simulink model "Modelo_benchmark"  (R2023a)
settings: Solver=VariableStepAuto  StartTime=0.0  StopTime=6250  RelTol=1e-3
values from neighbouring files (symbols this model uses):
  A = 0.0012    [control_temperatura.mat]    (also in var.m)
  C1_Q1 = 64.8931891795    [control_temperatura.mat]    (also in var.m = k3*Tau2)
  C1_Q2 = 0.0892445260493    [control_temperatura.mat]    (also in var.m = k1*k6)
  C2_Q1 = 0.558623321055    [control_temperatura.mat]    (also in var.m = k3)
  C_ff = GQ2T1cr/GQ1T1cr    [var.m]
  cp = 500    [control_temperatura.mat]    (also in var.m)
  e = zeros(1,iteraciones+ini)    [Codigo_discreto_ap.m]    (also in control_temperatura.mat = 0.9; var.m = 0.9)
  GQ1T1cr = tf(kcr1, [Taucr1 1])    [var.m]
  Hf1 = 0.01    [control_temperatura.mat]    (also in var.m)
  Hf2 = 0.004    [control_temperatura.mat]    (also in var.m)
  K_ap = 7.31538861094    [control_temperatura.mat]    (also in var.m = (2*delta*Taucr1*wn-1)/kcr1)
  K_cp = 1.15885597738    [control_temperatura.mat]    (also in var.m)
  m = 0.004    [control_temperatura.mat]    (also in var.m)
  P1_Q1 = 12978.6378359    [control_temperatura.mat]    (also in var.m = Tau1*Tau2)
  P1_Q2 = 12978.6378359    [control_temperatura.mat]    (also in var.m = Tau1*Tau2)
  P2_Q1 = 227.890937142    [control_temperatura.mat]    (also in var.m = Tau2+Tau1)
  P2_Q2 = 227.890937142    [control_temperatura.mat]    (also in var.m = Tau2+Tau1)
  P3_Q1 = 0.840856230771    [control_temperatura.mat]    (also in var.m = 1- k1*k4)
  P3_Q2 = 0.840856230771    [control_temperatura.mat]    (also in var.m = 1- k1*k4)
  T1i = 299.55    [control_temperatura.mat]    (also in var.m)
  T1o = 309.62355074    [control_temperatura.mat]    (also in var.m = x(1))
  T2i = 299.55    [control_temperatura.mat]    (also in var.m)
  TA = 299.55    [control_temperatura.mat]    (also in var.m)
  th = 5.67e-08    [control_temperatura.mat]    (also in var.m)
  Ti_ap = 23.6710802631    [control_temperatura.mat]    (also in var.m = (K_ap*kcr1)/(Taucr1*wn^2))
  Ti_cp = 165    [control_temperatura.mat]    (also in var.m)
  Tk = 273.15    [control_temperatura.mat]    (also in var.m)
  Tt_ap = 4.8652934406    [control_temperatura.mat]    (also in var.m = sqrt(Ti_ap))
  Tt_cp = 12.8452325787    [control_temperatura.mat]    (also in var.m = sqrt(Ti_cp))
  U = 1.4    [control_temperatura.mat]    (also in var.m)
undefined symbols (not defined in the file or in its folder): PID_Matlab
libraries: slpidlib x8, simulink_extras x6, simulink x4
(part 2 of 2)

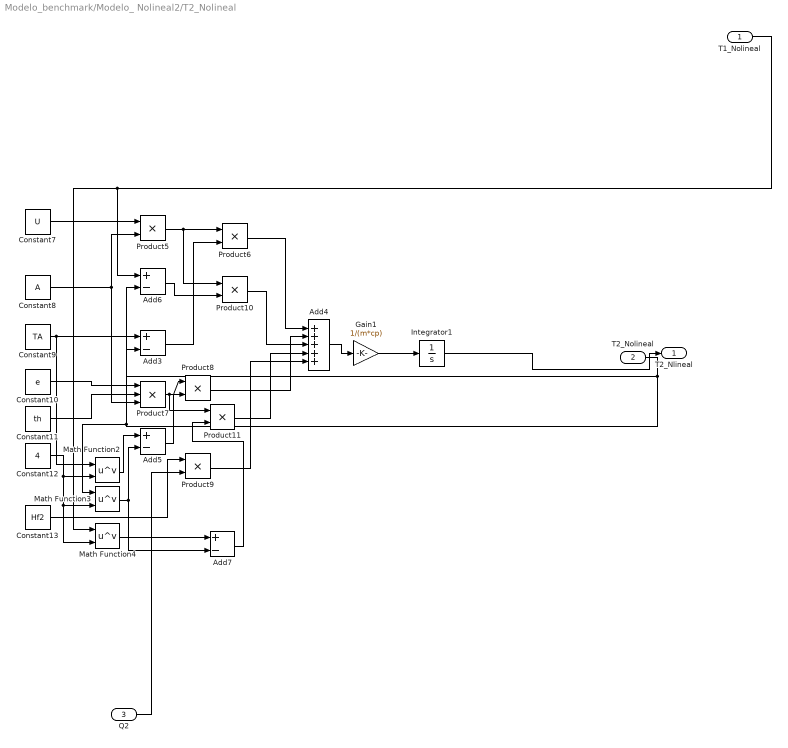
== system Modelo_benchmark/Modelo_ Nolineal2/T2_Nolineal ==
  T1_Nolineal : Inport
  T2_Nolineal : Inport  Port=2
  Q2 : Inport  Port=3
  Add{3,5..7} (4 alike) : Sum  Inputs=+-
  Add4 : Sum  Inputs=+++++
  Constant10 : Constant  Value=e
  Constant11 : Constant  Value=th
  Constant12 : Constant  Value=4
  Constant13 : Constant  Value=Hf2
  Constant7 : Constant  Value=U
  Constant8 : Constant  Value=A
  Constant9 : Constant  Value=TA
  Gain1 : Gain  Gain=1/(m*cp)
  Integrator1 : Integrator  InitialCondition=T2i
  Math Function2 : Math  Operator=pow
  Math Function3 : Math  Operator=pow
  Math Function4 : Math  Operator=pow
  Product{5..6,8..11} (6 alike) : Product
  Product7 : Product  Inputs=3
  T2_Nlineal : Outport
  wires:
  Integrator1/1 -> T2_Nlineal/1
  Product11/1 -> Add4/4
  T2_Nolineal/1 -> Add3/2, Math Function3/1, Add6/2
  Product7/1 -> Product11/1, Product8/1
  Constant7/1 -> Product5/1
  Product8/1 -> Add4/2
  T1_Nolineal/1 -> Math Function4/1, Add6/1
  Product9/1 -> Add4/5
  Math Function3/1 -> Add7/2, Add5/2
  Add6/1 -> Product10/2
  Add3/1 -> Product6/2
  Constant9/1 -> Math Function2/1, Add3/1
  Constant12/1 -> Math Function4/2, Math Function3/2, Math Function2/2
  Add4/1 -> Gain1/1
  Add5/1 -> Product8/2
  Constant11/1 -> Product7/2
  Constant13/1 -> Product9/1
  Gain1/1 -> Integrator1/1
  Constant8/1 -> Product5/2, Product7/3
  Product10/1 -> Add4/3
  Math Function4/1 -> Add7/1
  Math Function2/1 -> Add5/1
  Product6/1 -> Add4/1
  Q2/1 -> Product9/2
  Constant10/1 -> Product7/1
  Product5/1 -> Product10/1, Product6/1
  Add7/1 -> Product11/2

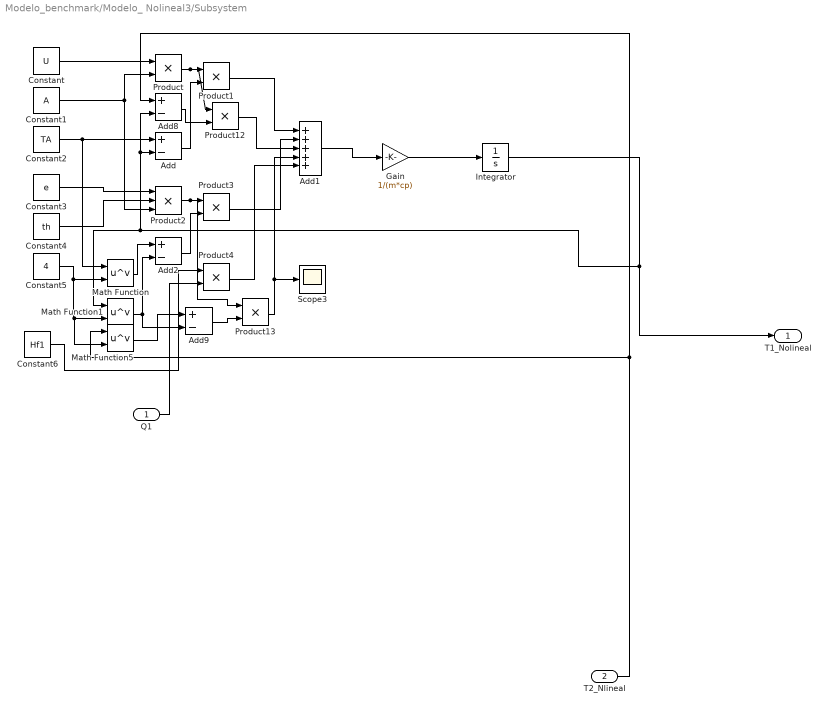
== system Modelo_benchmark/Modelo_ Nolineal3/Subsystem ==
  Q1 : Inport
  T2_Nlineal : Inport  Port=2
  Add{,2,8..9} (4 alike) : Sum  Inputs=+-
  Add1 : Sum  Inputs=+++++
  Constant : Constant  Value=U
  Constant1 : Constant  Value=A
  Constant2 : Constant  Value=TA
  Constant3 : Constant  Value=e
  Constant4 : Constant  Value=th
  Constant5 : Constant  Value=4
  Constant6 : Constant  Value=Hf1
  Gain : Gain  Gain=1/(m*cp)
  Integrator : Integrator  InitialCondition=T1i
  Math Function : Math  Operator=pow
  Math Function1 : Math  Operator=pow
  Math Function5 : Math  Operator=pow
  Product{,1,3..4,12..13} (6 alike) : Product
  Product2 : Product  Inputs=3
  Scope3 : Scope
  T1_Nolineal : Outport
  wires:
  Add/1 -> Product1/2
  Constant4/1 -> Product2/2
  Math Function5/1 -> Add9/1
  T2_Nlineal/1 -> Math Function5/1, Add8/1
  Product/1 -> Product12/1, Product1/1
  Constant3/1 -> Product2/1
  Math Function1/1 -> Add2/2, Add9/2
  Constant6/1 -> Product4/1
  Product3/1 -> Add1/2
  Product13/1 -> Scope3/1, Add1/4
  Product12/1 -> Add1/3
  Constant5/1 -> Math Function5/2, Math Function1/2, Math Function/2
  Constant1/1 -> Product2/3, Product/2
  Product1/1 -> Add1/1
  Constant/1 -> Product/1
  Gain/1 -> Integrator/1
  Constant2/1 -> Math Function/1, Add/1
  Product4/1 -> Add1/5
  Integrator/1 -> T1_Nolineal/1, Math Function1/1, Add8/2, Add/2
  Add2/1 -> Product3/2
  Add1/1 -> Gain/1
  Q1/1 -> Product4/2
  Product2/1 -> Product13/1, Product3/1
  Add8/1 -> Product12/2
  Math Function/1 -> Add2/1
  Add9/1 -> Product13/2

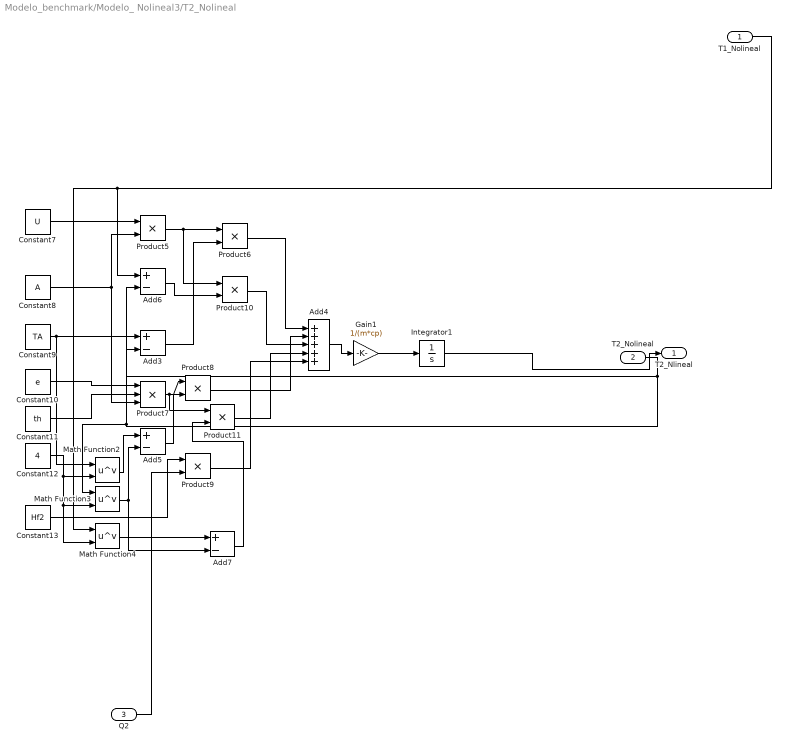
== system Modelo_benchmark/Modelo_ Nolineal3/T2_Nolineal ==
  T1_Nolineal : Inport
  T2_Nolineal : Inport  Port=2
  Q2 : Inport  Port=3
  Add{3,5..7} (4 alike) : Sum  Inputs=+-
  Add4 : Sum  Inputs=+++++
  Constant10 : Constant  Value=e
  Constant11 : Constant  Value=th
  Constant12 : Constant  Value=4
  Constant13 : Constant  Value=Hf2
  Constant7 : Constant  Value=U
  Constant8 : Constant  Value=A
  Constant9 : Constant  Value=TA
  Gain1 : Gain  Gain=1/(m*cp)
  Integrator1 : Integrator  InitialCondition=T2i
  Math Function2 : Math  Operator=pow
  Math Function3 : Math  Operator=pow
  Math Function4 : Math  Operator=pow
  Product{5..6,8..11} (6 alike) : Product
  Product7 : Product  Inputs=3
  T2_Nlineal : Outport
  wires:
  Integrator1/1 -> T2_Nlineal/1
  Product11/1 -> Add4/4
  T2_Nolineal/1 -> Add3/2, Math Function3/1, Add6/2
  Product7/1 -> Product11/1, Product8/1
  Constant7/1 -> Product5/1
  Product8/1 -> Add4/2
  T1_Nolineal/1 -> Math Function4/1, Add6/1
  Product9/1 -> Add4/5
  Math Function3/1 -> Add7/2, Add5/2
  Add6/1 -> Product10/2
  Add3/1 -> Product6/2
  Constant9/1 -> Math Function2/1, Add3/1
  Constant12/1 -> Math Function4/2, Math Function3/2, Math Function2/2
  Add4/1 -> Gain1/1
  Add5/1 -> Product8/2
  Constant11/1 -> Product7/2
  Constant13/1 -> Product9/1
  Gain1/1 -> Integrator1/1
  Constant8/1 -> Product5/2, Product7/3
  Product10/1 -> Add4/3
  Math Function4/1 -> Add7/1
  Math Function2/1 -> Add5/1
  Product6/1 -> Add4/1
  Q2/1 -> Product9/2
  Constant10/1 -> Product7/1
  Product5/1 -> Product10/1, Product6/1
  Add7/1 -> Product11/2

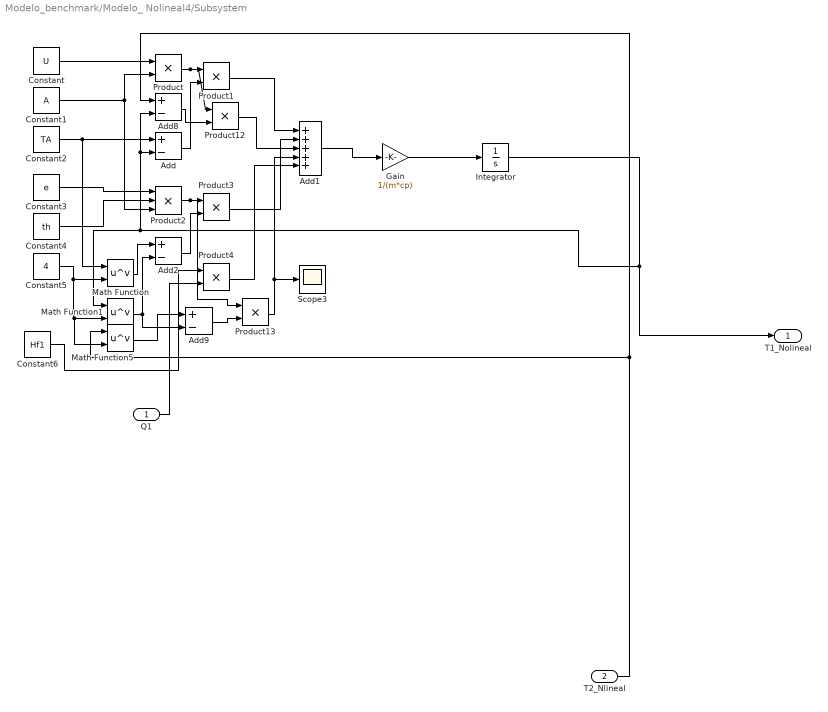
== system Modelo_benchmark/Modelo_ Nolineal4/Subsystem ==
  Q1 : Inport
  T2_Nlineal : Inport  Port=2
  Add{,2,8..9} (4 alike) : Sum  Inputs=+-
  Add1 : Sum  Inputs=+++++
  Constant : Constant  Value=U
  Constant1 : Constant  Value=A
  Constant2 : Constant  Value=TA
  Constant3 : Constant  Value=e
  Constant4 : Constant  Value=th
  Constant5 : Constant  Value=4
  Constant6 : Constant  Value=Hf1
  Gain : Gain  Gain=1/(m*cp)
  Integrator : Integrator  InitialCondition=T1i
  Math Function : Math  Operator=pow
  Math Function1 : Math  Operator=pow
  Math Function5 : Math  Operator=pow
  Product{,1,3..4,12..13} (6 alike) : Product
  Product2 : Product  Inputs=3
  Scope3 : Scope
  T1_Nolineal : Outport
  wires:
  Add/1 -> Product1/2
  Constant4/1 -> Product2/2
  Math Function5/1 -> Add9/1
  T2_Nlineal/1 -> Math Function5/1, Add8/1
  Product/1 -> Product12/1, Product1/1
  Constant3/1 -> Product2/1
  Math Function1/1 -> Add2/2, Add9/2
  Constant6/1 -> Product4/1
  Product3/1 -> Add1/2
  Product13/1 -> Scope3/1, Add1/4
  Product12/1 -> Add1/3
  Constant5/1 -> Math Function5/2, Math Function1/2, Math Function/2
  Constant1/1 -> Product2/3, Product/2
  Product1/1 -> Add1/1
  Constant/1 -> Product/1
  Gain/1 -> Integrator/1
  Constant2/1 -> Math Function/1, Add/1
  Product4/1 -> Add1/5
  Integrator/1 -> T1_Nolineal/1, Math Function1/1, Add8/2, Add/2
  Add2/1 -> Product3/2
  Add1/1 -> Gain/1
  Q1/1 -> Product4/2
  Product2/1 -> Product13/1, Product3/1
  Add8/1 -> Product12/2
  Math Function/1 -> Add2/1
  Add9/1 -> Product13/2

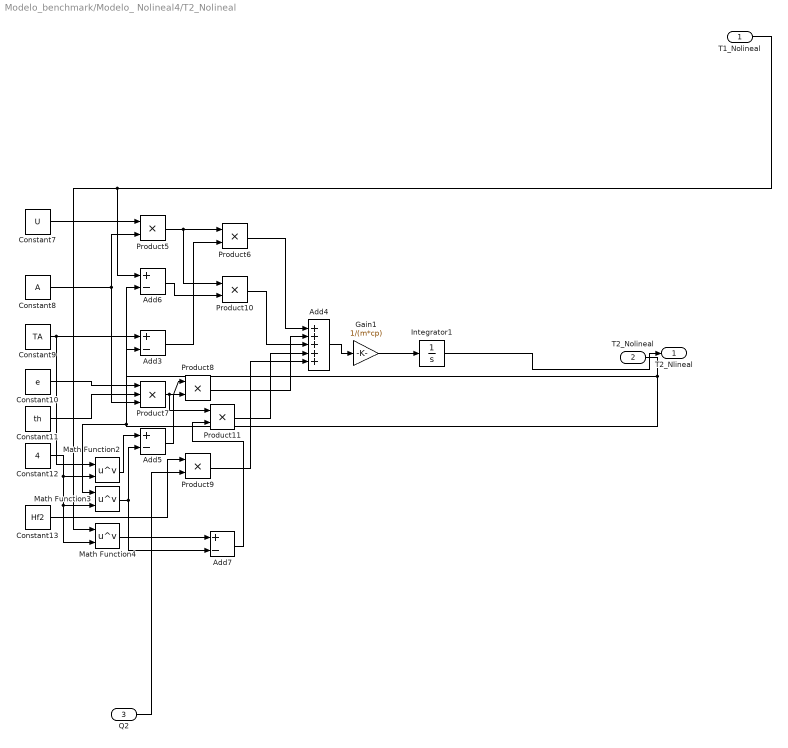
== system Modelo_benchmark/Modelo_ Nolineal4/T2_Nolineal ==
  T1_Nolineal : Inport
  T2_Nolineal : Inport  Port=2
  Q2 : Inport  Port=3
  Add{3,5..7} (4 alike) : Sum  Inputs=+-
  Add4 : Sum  Inputs=+++++
  Constant10 : Constant  Value=e
  Constant11 : Constant  Value=th
  Constant12 : Constant  Value=4
  Constant13 : Constant  Value=Hf2
  Constant7 : Constant  Value=U
  Constant8 : Constant  Value=A
  Constant9 : Constant  Value=TA
  Gain1 : Gain  Gain=1/(m*cp)
  Integrator1 : Integrator  InitialCondition=T2i
  Math Function2 : Math  Operator=pow
  Math Function3 : Math  Operator=pow
  Math Function4 : Math  Operator=pow
  Product{5..6,8..11} (6 alike) : Product
  Product7 : Product  Inputs=3
  T2_Nlineal : Outport
  wires:
  Integrator1/1 -> T2_Nlineal/1
  Product11/1 -> Add4/4
  T2_Nolineal/1 -> Add3/2, Math Function3/1, Add6/2
  Product7/1 -> Product11/1, Product8/1
  Constant7/1 -> Product5/1
  Product8/1 -> Add4/2
  T1_Nolineal/1 -> Math Function4/1, Add6/1
  Product9/1 -> Add4/5
  Math Function3/1 -> Add7/2, Add5/2
  Add6/1 -> Product10/2
  Add3/1 -> Product6/2
  Constant9/1 -> Math Function2/1, Add3/1
  Constant12/1 -> Math Function4/2, Math Function3/2, Math Function2/2
  Add4/1 -> Gain1/1
  Add5/1 -> Product8/2
  Constant11/1 -> Product7/2
  Constant13/1 -> Product9/1
  Gain1/1 -> Integrator1/1
  Constant8/1 -> Product5/2, Product7/3
  Product10/1 -> Add4/3
  Math Function4/1 -> Add7/1
  Math Function2/1 -> Add5/1
  Product6/1 -> Add4/1
  Q2/1 -> Product9/2
  Constant10/1 -> Product7/1
  Product5/1 -> Product10/1, Product6/1
  Add7/1 -> Product11/2

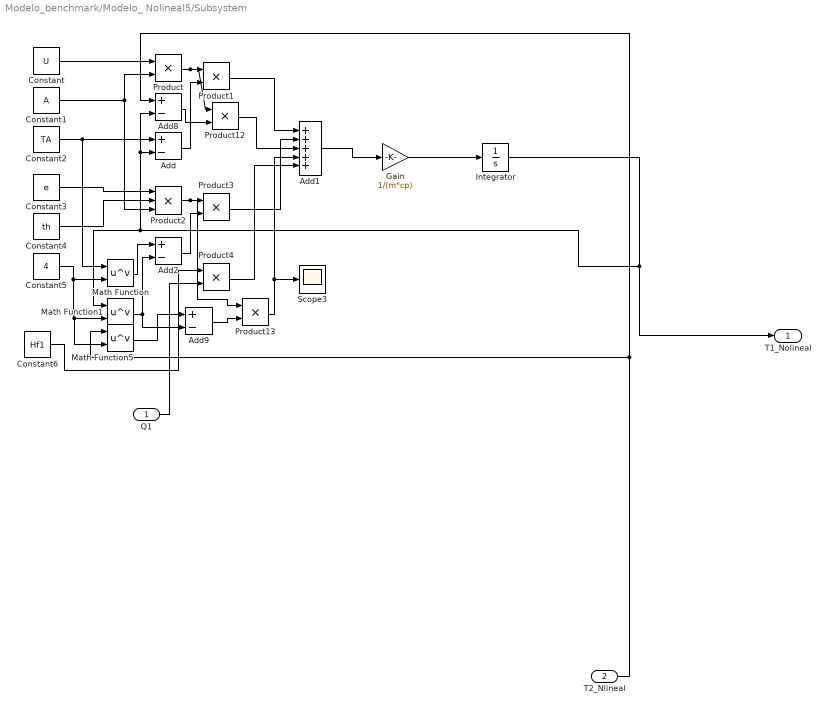
== system Modelo_benchmark/Modelo_ Nolineal5/Subsystem ==
  Q1 : Inport
  T2_Nlineal : Inport  Port=2
  Add{,2,8..9} (4 alike) : Sum  Inputs=+-
  Add1 : Sum  Inputs=+++++
  Constant : Constant  Value=U
  Constant1 : Constant  Value=A
  Constant2 : Constant  Value=TA
  Constant3 : Constant  Value=e
  Constant4 : Constant  Value=th
  Constant5 : Constant  Value=4
  Constant6 : Constant  Value=Hf1
  Gain : Gain  Gain=1/(m*cp)
  Integrator : Integrator  InitialCondition=T1i
  Math Function : Math  Operator=pow
  Math Function1 : Math  Operator=pow
  Math Function5 : Math  Operator=pow
  Product{,1,3..4,12..13} (6 alike) : Product
  Product2 : Product  Inputs=3
  Scope3 : Scope
  T1_Nolineal : Outport
  wires:
  Add/1 -> Product1/2
  Constant4/1 -> Product2/2
  Math Function5/1 -> Add9/1
  T2_Nlineal/1 -> Math Function5/1, Add8/1
  Product/1 -> Product12/1, Product1/1
  Constant3/1 -> Product2/1
  Math Function1/1 -> Add2/2, Add9/2
  Constant6/1 -> Product4/1
  Product3/1 -> Add1/2
  Product13/1 -> Scope3/1, Add1/4
  Product12/1 -> Add1/3
  Constant5/1 -> Math Function5/2, Math Function1/2, Math Function/2
  Constant1/1 -> Product2/3, Product/2
  Product1/1 -> Add1/1
  Constant/1 -> Product/1
  Gain/1 -> Integrator/1
  Constant2/1 -> Math Function/1, Add/1
  Product4/1 -> Add1/5
  Integrator/1 -> T1_Nolineal/1, Math Function1/1, Add8/2, Add/2
  Add2/1 -> Product3/2
  Add1/1 -> Gain/1
  Q1/1 -> Product4/2
  Product2/1 -> Product13/1, Product3/1
  Add8/1 -> Product12/2
  Math Function/1 -> Add2/1
  Add9/1 -> Product13/2

== system Modelo_benchmark/Modelo_ Nolineal5/T2_Nolineal ==
  T1_Nolineal : Inport
  T2_Nolineal : Inport  Port=2
  Q2 : Inport  Port=3
  Add{3,5..7} (4 alike) : Sum  Inputs=+-
  Add4 : Sum  Inputs=+++++
  Constant10 : Constant  Value=e
  Constant11 : Constant  Value=th
  Constant12 : Constant  Value=4
  Constant13 : Constant  Value=Hf2
  Constant7 : Constant  Value=U
  Constant8 : Constant  Value=A
  Constant9 : Constant  Value=TA
  Gain1 : Gain  Gain=1/(m*cp)
  Integrator1 : Integrator  InitialCondition=T2i
  Math Function2 : Math  Operator=pow
  Math Function3 : Math  Operator=pow
  Math Function4 : Math  Operator=pow
  Product{5..6,8..11} (6 alike) : Product
  Product7 : Product  Inputs=3
  T2_Nlineal : Outport
  wires:
  Integrator1/1 -> T2_Nlineal/1
  Product11/1 -> Add4/4
  T2_Nolineal/1 -> Add3/2, Math Function3/1, Add6/2
  Product7/1 -> Product11/1, Product8/1
  Constant7/1 -> Product5/1
  Product8/1 -> Add4/2
  T1_Nolineal/1 -> Math Function4/1, Add6/1
  Product9/1 -> Add4/5
  Math Function3/1 -> Add7/2, Add5/2
  Add6/1 -> Product10/2
  Add3/1 -> Product6/2
  Constant9/1 -> Math Function2/1, Add3/1
  Constant12/1 -> Math Function4/2, Math Function3/2, Math Function2/2
  Add4/1 -> Gain1/1
  Add5/1 -> Product8/2
  Constant11/1 -> Product7/2
  Constant13/1 -> Product9/1
  Gain1/1 -> Integrator1/1
  Constant8/1 -> Product5/2, Product7/3
  Product10/1 -> Add4/3
  Math Function4/1 -> Add7/1
  Math Function2/1 -> Add5/1
  Product6/1 -> Add4/1
  Q2/1 -> Product9/2
  Constant10/1 -> Product7/1
  Product5/1 -> Product10/1, Product6/1
  Add7/1 -> Product11/2

== system Modelo_benchmark/Modelo_ Nolineal6/Subsystem ==
  Q1 : Inport
  T2_Nlineal : Inport  Port=2
  Add{,2,8..9} (4 alike) : Sum  Inputs=+-
  Add1 : Sum  Inputs=+++++
  Constant : Constant  Value=U
  Constant1 : Constant  Value=A
  Constant2 : Constant  Value=TA
  Constant3 : Constant  Value=e
  Constant4 : Constant  Value=th
  Constant5 : Constant  Value=4
  Constant6 : Constant  Value=Hf1
  Gain : Gain  Gain=1/(m*cp)
  Integrator : Integrator  InitialCondition=T1i
  Math Function : Math  Operator=pow
  Math Function1 : Math  Operator=pow
  Math Function5 : Math  Operator=pow
  Product{,1,3..4,12..13} (6 alike) : Product
  Product2 : Product  Inputs=3
  Scope3 : Scope
  T1_Nolineal : Outport
  wires:
  Add/1 -> Product1/2
  Constant4/1 -> Product2/2
  Math Function5/1 -> Add9/1
  T2_Nlineal/1 -> Math Function5/1, Add8/1
  Product/1 -> Product12/1, Product1/1
  Constant3/1 -> Product2/1
  Math Function1/1 -> Add2/2, Add9/2
  Constant6/1 -> Product4/1
  Product3/1 -> Add1/2
  Product13/1 -> Scope3/1, Add1/4
  Product12/1 -> Add1/3
  Constant5/1 -> Math Function5/2, Math Function1/2, Math Function/2
  Constant1/1 -> Product2/3, Product/2
  Product1/1 -> Add1/1
  Constant/1 -> Product/1
  Gain/1 -> Integrator/1
  Constant2/1 -> Math Function/1, Add/1
  Product4/1 -> Add1/5
  Integrator/1 -> T1_Nolineal/1, Math Function1/1, Add8/2, Add/2
  Add2/1 -> Product3/2
  Add1/1 -> Gain/1
  Q1/1 -> Product4/2
  Product2/1 -> Product13/1, Product3/1
  Add8/1 -> Product12/2
  Math Function/1 -> Add2/1
  Add9/1 -> Product13/2

== system Modelo_benchmark/Modelo_ Nolineal6/T2_Nolineal ==
  T1_Nolineal : Inport
  T2_Nolineal : Inport  Port=2
  Q2 : Inport  Port=3
  Add{3,5..7} (4 alike) : Sum  Inputs=+-
  Add4 : Sum  Inputs=+++++
  Constant10 : Constant  Value=e
  Constant11 : Constant  Value=th
  Constant12 : Constant  Value=4
  Constant13 : Constant  Value=Hf2
  Constant7 : Constant  Value=U
  Constant8 : Constant  Value=A
  Constant9 : Constant  Value=TA
  Gain1 : Gain  Gain=1/(m*cp)
  Integrator1 : Integrator  InitialCondition=T2i
  Math Function2 : Math  Operator=pow
  Math Function3 : Math  Operator=pow
  Math Function4 : Math  Operator=pow
  Product{5..6,8..11} (6 alike) : Product
  Product7 : Product  Inputs=3
  T2_Nlineal : Outport
  wires:
  Integrator1/1 -> T2_Nlineal/1
  Product11/1 -> Add4/4
  T2_Nolineal/1 -> Add3/2, Math Function3/1, Add6/2
  Product7/1 -> Product11/1, Product8/1
  Constant7/1 -> Product5/1
  Product8/1 -> Add4/2
  T1_Nolineal/1 -> Math Function4/1, Add6/1
  Product9/1 -> Add4/5
  Math Function3/1 -> Add7/2, Add5/2
  Add6/1 -> Product10/2
  Add3/1 -> Product6/2
  Constant9/1 -> Math Function2/1, Add3/1
  Constant12/1 -> Math Function4/2, Math Function3/2, Math Function2/2
  Add4/1 -> Gain1/1
  Add5/1 -> Product8/2
  Constant11/1 -> Product7/2
  Constant13/1 -> Product9/1
  Gain1/1 -> Integrator1/1
  Constant8/1 -> Product5/2, Product7/3
  Product10/1 -> Add4/3
  Math Function4/1 -> Add7/1
  Math Function2/1 -> Add5/1
  Product6/1 -> Add4/1
  Q2/1 -> Product9/2
  Constant10/1 -> Product7/1
  Product5/1 -> Product10/1, Product6/1
  Add7/1 -> Product11/2
